simulink model "TST_OilP_VD"  (R2016b)
settings: Solver=FixedStepDiscrete  StartTime=0.0  StopTime=simTime  FixedStep=sampleTime  RelTol=1e-3
values from neighbouring files (symbols this model uses):
  testCase = 1    [initTST_OilP_VD_001.m]
libraries: simulink x4, UnitTest_Lib x2
settings Model: Creator=xinchangran  LastModifiedBy=xinchangran
settings DebuggingCC: SignalRangeChecking=error

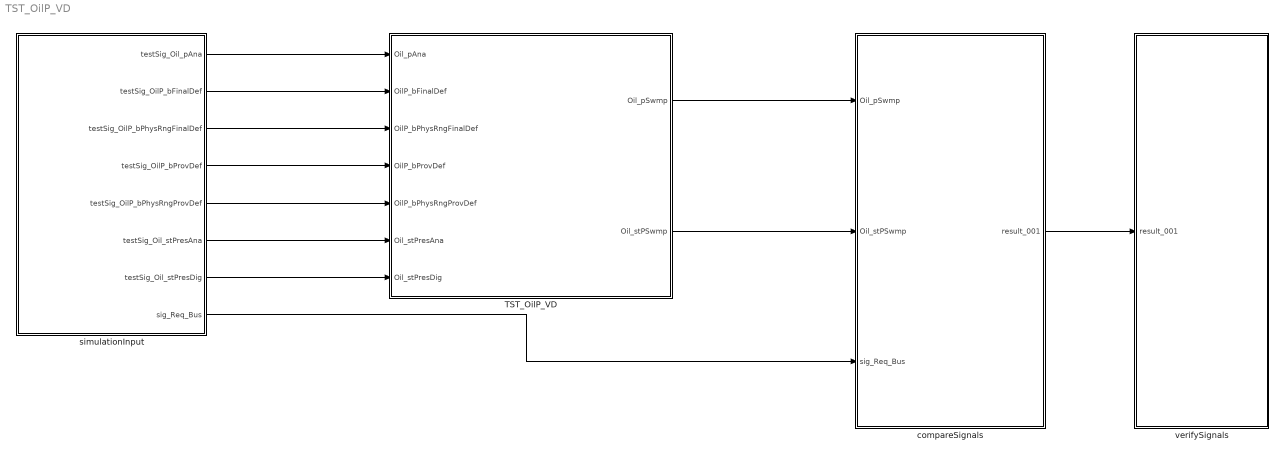
== system TST_OilP_VD ==
  TST_OilP_VD : Subsystem
  compareSignals : Subsystem
  simulationInput : Subsystem
  verifySignals : Subsystem
  wires:
  simulationInput/1(testSig_Oil_pAna) -> TST_OilP_VD/1(Oil_pAna)
  simulationInput/2(testSig_OilP_bFinalDef) -> TST_OilP_VD/2(OilP_bFinalDef)
  simulationInput/3(testSig_OilP_bPhysRngFinalDef) -> TST_OilP_VD/3(OilP_bPhysRngFinalDef)
  simulationInput/4(testSig_OilP_bProvDef) -> TST_OilP_VD/4(OilP_bProvDef)
  simulationInput/5(testSig_OilP_bPhysRngProvDef) -> TST_OilP_VD/5(OilP_bPhysRngProvDef)
  simulationInput/6(testSig_Oil_stPresAna) -> TST_OilP_VD/6(Oil_stPresAna)
  simulationInput/7(testSig_Oil_stPresDig) -> TST_OilP_VD/7(Oil_stPresDig)
  TST_OilP_VD/1(Oil_pSwmp) -> compareSignals/1(Oil_pSwmp)
  TST_OilP_VD/2(Oil_stPSwmp) -> compareSignals/2(Oil_stPSwmp)
  simulationInput/8(sig_Req_Bus) -> compareSignals/3(sig_Req_Bus)
  compareSignals/1(result_001) -> verifySignals/1(result_001)

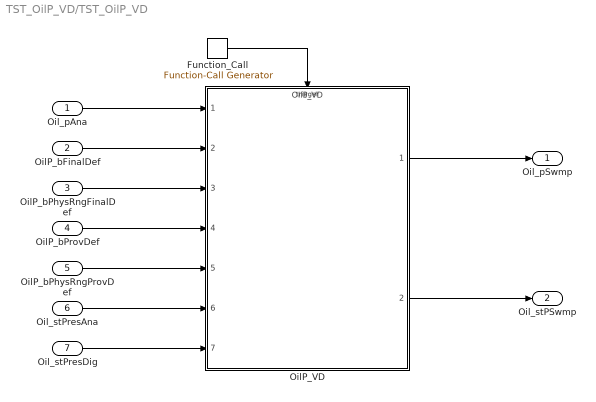
== system TST_OilP_VD/TST_OilP_VD ==
  Oil_pAna : Inport
  OilP_bFinalDef : Inport  Port=2
  OilP_bPhysRngFinalDef : Inport  Port=3
  OilP_bProvDef : Inport  Port=4
  OilP_bPhysRngProvDef : Inport  Port=5
  Oil_stPresAna : Inport  Port=6
  Oil_stPresDig : Inport  Port=7
  Function_Call : simulink/Ports & Subsystems/Function-Call Generator  sample_time=sampleTime  numberOfIterations=1
  OilP_VD : ModelReference  ModelNameDialog=OilP_VD  SimulationMode=Normal  ModelReferenceVersion=1.22  TriggerPortName=function  TriggerPortTriggerType=function-call  TriggerPortStatesWhenEnabling=held
  Oil_pSwmp : Outport
  Oil_stPSwmp : Outport  Port=2
  wires:
  Function_Call/1 -> OilP_VD/Trigger
  Oil_pAna/1 -> OilP_VD/1
  OilP_bFinalDef/1 -> OilP_VD/2
  OilP_bPhysRngFinalDef/1 -> OilP_VD/3
  OilP_bProvDef/1 -> OilP_VD/4
  OilP_bPhysRngProvDef/1 -> OilP_VD/5
  Oil_stPresAna/1 -> OilP_VD/6
  Oil_stPresDig/1 -> OilP_VD/7
  OilP_VD/1 -> Oil_pSwmp/1
  OilP_VD/2 -> Oil_stPSwmp/1

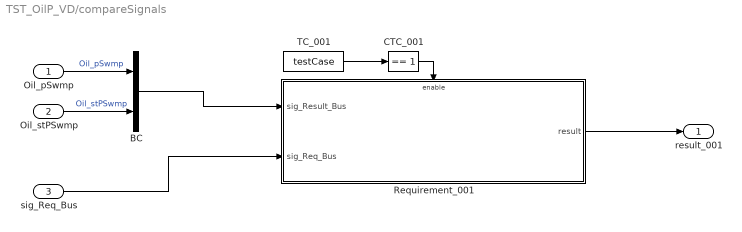
== system TST_OilP_VD/compareSignals ==
  Oil_pSwmp : Inport
  Oil_stPSwmp : Inport  Port=2
  sig_Req_Bus : Inport  Port=3
  BC : BusCreator  Inputs=2
  CTC_001 : simulink/Logic and Bit Operations/Compare To Constant  relop===  const=1  OutDataTypeStr=boolean
  Requirement_001 : Subsystem
  TC_001 : Constant  Value=testCase
  result_001 : Outport
  wires:
  Oil_pSwmp/1 -> BC/1  "Oil_pSwmp"
  Oil_stPSwmp/1 -> BC/2  "Oil_stPSwmp"
  TC_001/1 -> CTC_001/1
  CTC_001/1 -> Requirement_001/Enable
  sig_Req_Bus/1 -> Requirement_001/2(sig_Req_Bus)
  BC/1 -> Requirement_001/1(sig_Result_Bus)
  Requirement_001/1(result) -> result_001/1

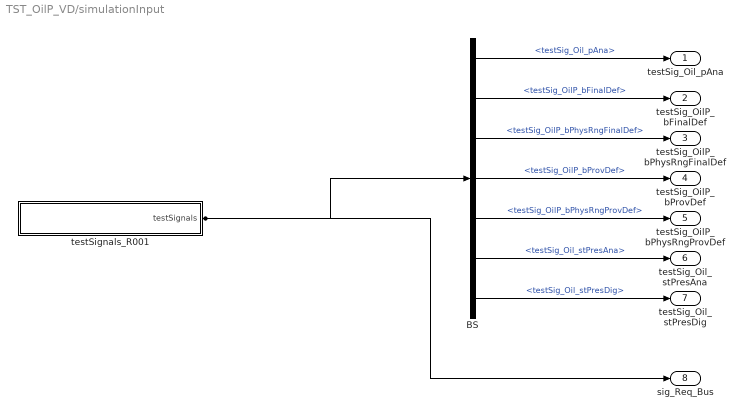
== system TST_OilP_VD/simulationInput ==
  BS : BusSelector  OutputSignals=testSig_Oil_pAna,testSig_OilP_bFinalDef,testSig_OilP_bPhysRngFinalDef,testSig_OilP_bProvDef,testSig_OilP_bPhysRngProvDef,testSig_Oil_stPresAna,testSig_Oil_stPresDig
  testSignals_R001 : Subsystem
  testSig_Oil_pAna : Outport
  testSig_OilP_bFinalDef : Outport  Port=2
  testSig_OilP_bPhysRngFinalDef : Outport  Port=3
  testSig_OilP_bProvDef : Outport  Port=4
  testSig_OilP_bPhysRngProvDef : Outport  Port=5
  testSig_Oil_stPresAna : Outport  Port=6
  testSig_Oil_stPresDig : Outport  Port=7
  sig_Req_Bus : Outport  Port=8
  wires:
  BS/1 -> testSig_Oil_pAna/1  "<testSig_Oil_pAna>"
  BS/2 -> testSig_OilP_bFinalDef/1  "<testSig_OilP_bFinalDef>"
  BS/3 -> testSig_OilP_bPhysRngFinalDef/1  "<testSig_OilP_bPhysRngFinalDef>"
  BS/4 -> testSig_OilP_bProvDef/1  "<testSig_OilP_bProvDef>"
  BS/5 -> testSig_OilP_bPhysRngProvDef/1  "<testSig_OilP_bPhysRngProvDef>"
  BS/6 -> testSig_Oil_stPresAna/1  "<testSig_Oil_stPresAna>"
  BS/7 -> testSig_Oil_stPresDig/1  "<testSig_Oil_stPresDig>"
  testSignals_R001/1(testSignals) -> BS/1, sig_Req_Bus/1

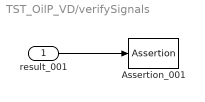
== system TST_OilP_VD/verifySignals ==
  result_001 : Inport
  Assertion_001 : Assertion  Enabled=off
  wires:
  result_001/1 -> Assertion_001/1

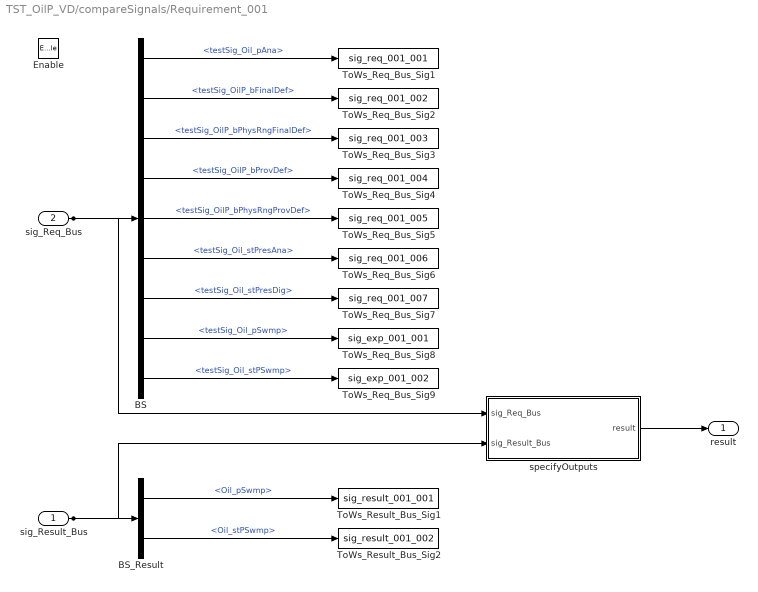
== system TST_OilP_VD/compareSignals/Requirement_001 ==
  sig_Result_Bus : Inport
  sig_Req_Bus : Inport  Port=2
  Enable : EnablePort
  BS : BusSelector  OutputSignals=testSig_Oil_pAna,testSig_OilP_bFinalDef,testSig_OilP_bPhysRngFinalDef,testSig_OilP_bProvDef,testSig_OilP_bPhysRngProvDef,testSig_Oil_stPresAna,testSig_Oil_stPresDig,testSig_Oil_pSwmp,testSig_Oil_stPSwmp
  BS_Result : BusSelector  OutputSignals=Oil_pSwmp,Oil_stPSwmp
  ToWs_Req_Bus_Sig1 : ToWorkspace  VariableName=sig_req_001_001  SaveFormat=Structure With Time
  ToWs_Req_Bus_Sig2 : ToWorkspace  VariableName=sig_req_001_002  SaveFormat=Structure With Time
  ToWs_Req_Bus_Sig3 : ToWorkspace  VariableName=sig_req_001_003  SaveFormat=Structure With Time
  ToWs_Req_Bus_Sig4 : ToWorkspace  VariableName=sig_req_001_004  SaveFormat=Structure With Time
  ToWs_Req_Bus_Sig5 : ToWorkspace  VariableName=sig_req_001_005  SaveFormat=Structure With Time
  ToWs_Req_Bus_Sig6 : ToWorkspace  VariableName=sig_req_001_006  SaveFormat=Structure With Time
  ToWs_Req_Bus_Sig7 : ToWorkspace  VariableName=sig_req_001_007  SaveFormat=Structure With Time
  ToWs_Req_Bus_Sig8 : ToWorkspace  VariableName=sig_exp_001_001  SaveFormat=Structure With Time
  ToWs_Req_Bus_Sig9 : ToWorkspace  VariableName=sig_exp_001_002  SaveFormat=Structure With Time
  ToWs_Result_Bus_Sig1 : ToWorkspace  VariableName=sig_result_001_001  SaveFormat=Structure With Time
  ToWs_Result_Bus_Sig2 : ToWorkspace  VariableName=sig_result_001_002  SaveFormat=Structure With Time
  specifyOutputs : Subsystem
  result : Outport
  wires:
  sig_Req_Bus/1 -> BS/1, specifyOutputs/1(sig_Req_Bus)
  BS/1 -> ToWs_Req_Bus_Sig1/1  "<testSig_Oil_pAna>"
  BS/2 -> ToWs_Req_Bus_Sig2/1  "<testSig_OilP_bFinalDef>"
  BS/3 -> ToWs_Req_Bus_Sig3/1  "<testSig_OilP_bPhysRngFinalDef>"
  BS/4 -> ToWs_Req_Bus_Sig4/1  "<testSig_OilP_bProvDef>"
  BS/5 -> ToWs_Req_Bus_Sig5/1  "<testSig_OilP_bPhysRngProvDef>"
  BS/6 -> ToWs_Req_Bus_Sig6/1  "<testSig_Oil_stPresAna>"
  BS/7 -> ToWs_Req_Bus_Sig7/1  "<testSig_Oil_stPresDig>"
  BS/8 -> ToWs_Req_Bus_Sig8/1  "<testSig_Oil_pSwmp>"
  BS/9 -> ToWs_Req_Bus_Sig9/1  "<testSig_Oil_stPSwmp>"
  sig_Result_Bus/1 -> BS_Result/1, specifyOutputs/2(sig_Result_Bus)
  BS_Result/1 -> ToWs_Result_Bus_Sig1/1  "<Oil_pSwmp>"
  BS_Result/2 -> ToWs_Result_Bus_Sig2/1  "<Oil_stPSwmp>"
  specifyOutputs/1(result) -> result/1

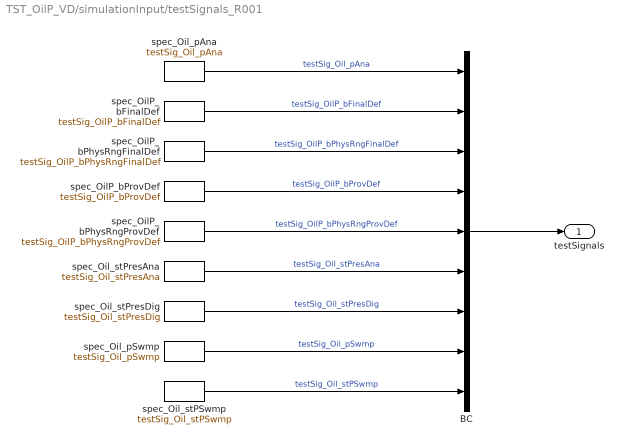
== system TST_OilP_VD/simulationInput/testSignals_R001 ==
  BC : BusCreator  Inputs=9
  spec_OilP_bFinalDef : FromWorkspace  VariableName=testSig_OilP_bFinalDef  Interpolate=off  OutputAfterFinalValue=Holding final value
  spec_OilP_bPhysRngFinalDef : FromWorkspace  VariableName=testSig_OilP_bPhysRngFinalDef  Interpolate=off  OutputAfterFinalValue=Holding final value
  spec_OilP_bPhysRngProvDef : FromWorkspace  VariableName=testSig_OilP_bPhysRngProvDef  Interpolate=off  OutputAfterFinalValue=Holding final value
  spec_OilP_bProvDef : FromWorkspace  VariableName=testSig_OilP_bProvDef  Interpolate=off  OutputAfterFinalValue=Holding final value
  spec_Oil_pAna : FromWorkspace  VariableName=testSig_Oil_pAna  Interpolate=off  OutputAfterFinalValue=Holding final value
  spec_Oil_pSwmp : FromWorkspace  VariableName=testSig_Oil_pSwmp  Interpolate=off  OutputAfterFinalValue=Holding final value
  spec_Oil_stPSwmp : FromWorkspace  VariableName=testSig_Oil_stPSwmp  Interpolate=off  OutputAfterFinalValue=Holding final value
  spec_Oil_stPresAna : FromWorkspace  VariableName=testSig_Oil_stPresAna  Interpolate=off  OutputAfterFinalValue=Holding final value
  spec_Oil_stPresDig : FromWorkspace  VariableName=testSig_Oil_stPresDig  Interpolate=off  OutputAfterFinalValue=Holding final value
  testSignals : Outport
  wires:
  BC/1 -> testSignals/1
  spec_Oil_pAna/1 -> BC/1  "testSig_Oil_pAna"
  spec_OilP_bFinalDef/1 -> BC/2  "testSig_OilP_bFinalDef"
  spec_OilP_bPhysRngFinalDef/1 -> BC/3  "testSig_OilP_bPhysRngFinalDef"
  spec_OilP_bProvDef/1 -> BC/4  "testSig_OilP_bProvDef"
  spec_OilP_bPhysRngProvDef/1 -> BC/5  "testSig_OilP_bPhysRngProvDef"
  spec_Oil_stPresAna/1 -> BC/6  "testSig_Oil_stPresAna"
  spec_Oil_stPresDig/1 -> BC/7  "testSig_Oil_stPresDig"
  spec_Oil_pSwmp/1 -> BC/8  "testSig_Oil_pSwmp"
  spec_Oil_stPSwmp/1 -> BC/9  "testSig_Oil_stPSwmp"

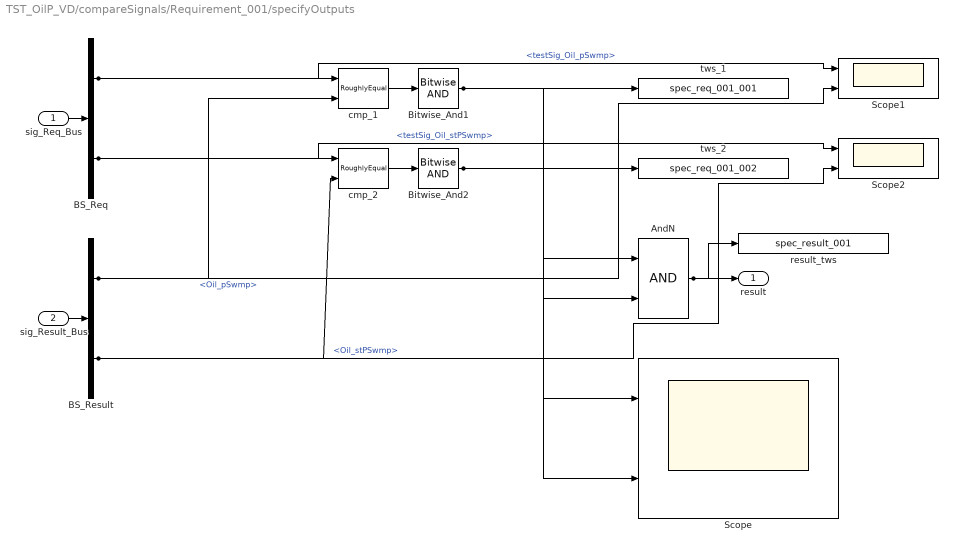
== system TST_OilP_VD/compareSignals/Requirement_001/specifyOutputs ==
  sig_Req_Bus : Inport
  sig_Result_Bus : Inport  Port=2
  AndN : Logic
  BS_Req : BusSelector  OutputSignals=testSig_Oil_pSwmp,testSig_Oil_stPSwmp
  BS_Result : BusSelector  OutputSignals=Oil_pSwmp,Oil_stPSwmp
  Bitwise_And1 : simulink/Logic and Bit Operations/Bitwise Operator  logicop=AND  UseBitMask=off  BitMask=bin2dec('11011001')  BitMaskRealWorld=Stored Integer
  Bitwise_And2 : simulink/Logic and Bit Operations/Bitwise Operator  logicop=AND  UseBitMask=off  BitMask=bin2dec('11011001')  BitMaskRealWorld=Stored Integer
  Scope : Scope  NumInputPorts=2
  Scope1 : Scope  NumInputPorts=2
  Scope2 : Scope  NumInputPorts=2
  cmp_1 : UnitTest_Lib/RoughlyEqual  slope=0.1
  cmp_2 : UnitTest_Lib/RoughlyEqual  slope=0.1
  result_tws : ToWorkspace  VariableName=spec_result_001
  tws_1 : ToWorkspace  VariableName=spec_req_001_001
  tws_2 : ToWorkspace  VariableName=spec_req_001_002
  result : Outport
  wires:
  sig_Req_Bus/1 -> BS_Req/1
  sig_Result_Bus/1 -> BS_Result/1
  AndN/1 -> result/1, result_tws/1
  BS_Req/1 -> cmp_1/1, Scope1/1  "<testSig_Oil_pSwmp>"
  BS_Result/1 -> cmp_1/2, Scope1/2  "<Oil_pSwmp>"
  cmp_1/1 -> Bitwise_And1/1
  Bitwise_And1/1 -> tws_1/1, AndN/1, Scope/1
  BS_Req/2 -> cmp_2/1, Scope2/1  "<testSig_Oil_stPSwmp>"
  BS_Result/2 -> cmp_2/2, Scope2/2  "<Oil_stPSwmp>"
  cmp_2/1 -> Bitwise_And2/1
  Bitwise_And2/1 -> tws_2/1, AndN/2, Scope/2
